simulink model "sampleModel305"  (R2021b)
settings: Solver=VariableStepAuto  StartTime=0.0  StopTime=10.0  RelTol=1e-3
libraries: simulink x7, slpidlib x1
settings Model: Creator=user  LastModifiedBy=user

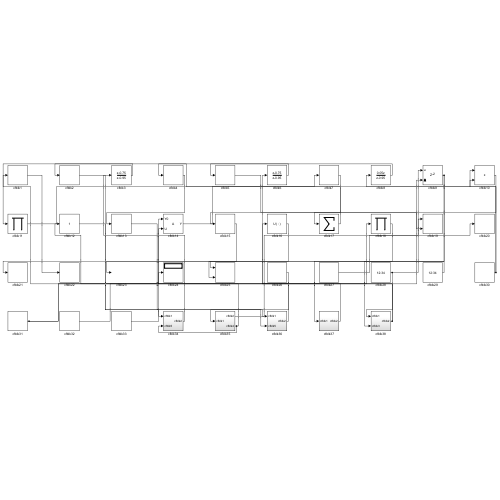
[thumbnail: Simulink's stored preview of the top-level diagram]
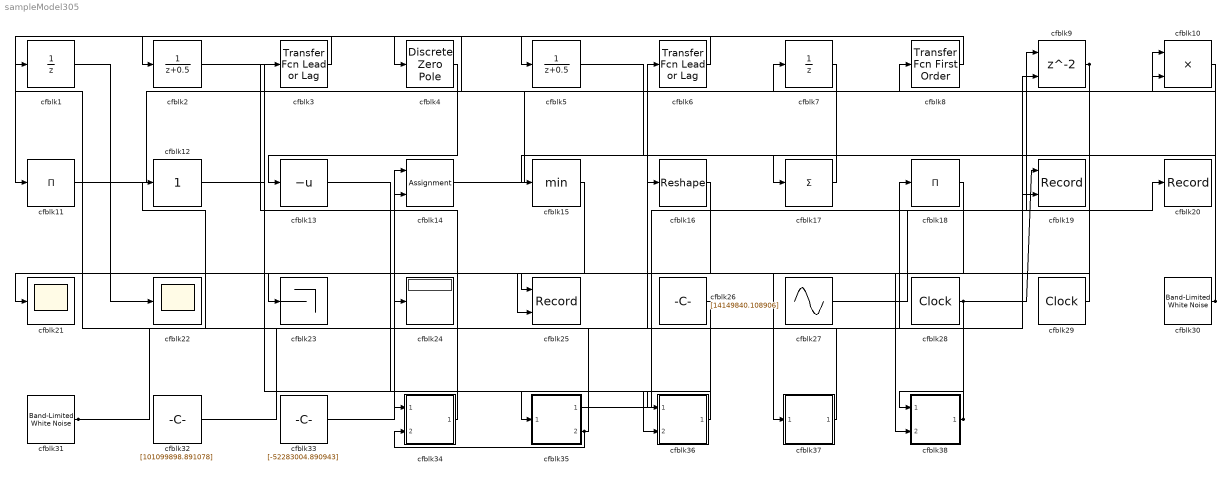
== system sampleModel305 ==
  cfblk1 : UnitDelay  HasFrameUpgradeWarning=on
  cfblk10 : Product  Inputs=**
  cfblk11 : Product  Inputs=*
  cfblk12 : simulink/Math Operations/Slider Gain  gain=1  low=0  high=2
  cfblk13 : UnaryMinus
  cfblk14 : Assignment  DiagnosticForDimensions=Warning  IndexOptions=Index vector (dialog)  Indices=1  OutputSizes=1
  cfblk15 : MinMax
  cfblk16 : Reshape
  cfblk17 : Sum  Inputs=+
  cfblk18 : Product  Inputs=*
  cfblk19 : Record  FileSettingsInternal="{\"entries\":[{\"content\":{\"excelSettings\":{\"content\":{},\"type\":\"Streamout.ExcelSettings\"}},\"type\":\"Streamout.FileSettingStorage\",\"uuid\":\"63984bb0-c559-4448-9fc6-104896ff0659\"}],\"packageUris\":[\"http://schema.mathworks.com/mf0/streamout_blocks/R2020a\"],\"version\":\"1.0\"}"  Layout=[1 1]  SignalsInternal="{\"entries\":[{\"content\":{\"signals\":[{\"content\":{\"blockPath\":[\"sampleModel305/cfblk19\"],\"channel\":[],\"dimensions\":[1],\"domain\":\"sampleModel305/cfblk19\",\"lineColor\":\"#a2142f\",\"plots\":[1],\"port\":1,\"sid\":[\"\"],\"signalID\":13014,\"signalName\":\"cfblk28\"},\"type\":\"RecordBlkView.Signal\",\"uuid\":\"141cd215-84be-4e50-999d-5b1fe4f06e84\"},{\"content\":{\"blockPath\":[\"sampleModel305/cfblk19\"],\"channel\":[],\"dimensions\":[1],\"domain\":\"sampleModel305/cfblk19\",\"lineColor\":\"#139fff\",\"plots\":[1],\"port\":2,\"sid\":[\"\"],\"signalID\":13018,\"signalName\":\"cfblk5\"},\"type\":\"RecordBlkView.Signal\",\"uuid\":\"dcc0499d-3265-4208-832f-2459034609dc\"}]},\"type\":\"RecordBlkView.InputSignals\",\"uuid\":\"7f0c9375-5767-4acb-9abc-590f8e22dae8\"}],\"packageUris\":[\"http://schema.mathworks.com/mf0/streamout_blocks/R2020a\"],\"version\":\"1.0\"}"  VisualizationBindings="{\"xyplotplugin\":{\"info\":[{\"series\":[{\"bindingParametersList\":[{\"parameter\":\"X-Axis\",\"signalID\":13014,\"signalName\":\"cfblk28\"},{\"parameter\":\"Y-Axis\",\"signalID\":13018,\"signalName\":\"cfblk5\"}],\"seriesID\":43943}],\"subplotID\":1}]}}"  CompatibilityTag=XY
  cfblk2 : DiscreteTransferFcn  SampleTime=1
  cfblk20 : Record  FileSettingsInternal="{\"entries\":[{\"content\":{\"excelSettings\":{\"content\":{},\"type\":\"Streamout.ExcelSettings\"}},\"type\":\"Streamout.FileSettingStorage\",\"uuid\":\"fa745143-092b-49d5-8c77-bd1d4f02d415\"}],\"packageUris\":[\"http://schema.mathworks.com/mf0/streamout_blocks/R2020a\"],\"version\":\"1.0\"}"  SignalsInternal="{\"entries\":[{\"content\":{\"signals\":[{\"content\":{\"blockPath\":[\"sampleModel305/cfblk20\"],\"channel\":[],\"dimensions\":[1],\"domain\":\"sampleModel305/cfblk20\",\"lineColor\":\"#7e2f8e\",\"plots\":[1],\"port\":1,\"sid\":[\"\"],\"signalID\":13030,\"signalName\":\"cfblk27\"},\"type\":\"RecordBlkView.Signal\",\"uuid\":\"72bc61b7-b3db-4e59-b8bd-afabd6830a11\"}]},\"type\":\"RecordBlkView.InputSignals\",\"uuid\":\"cfa96d27-1d36-46cd-bd3b-7bc137c001bd\"}],\"packageUris\":[\"http://schema.mathworks.com/mf0/streamout_blocks/R2020a\"],\"version\":\"1.0\"}"  VisualizationBindings="{\"sparklinesplugin\":{\"info\":[{\"bindingParametersList\":[],\"subplotID\":1}]}}"
  cfblk21 : Scope
  cfblk22 : Scope
  cfblk23 : Terminator
  cfblk24 : Display
  cfblk25 : Record  FileSettingsInternal="{\"entries\":[{\"content\":{\"excelSettings\":{\"content\":{},\"type\":\"Streamout.ExcelSettings\"}},\"type\":\"Streamout.FileSettingStorage\",\"uuid\":\"4ed7394e-1e80-4f63-a180-05586a1c6fb6\"}],\"packageUris\":[\"http://schema.mathworks.com/mf0/streamout_blocks/R2020a\"],\"version\":\"1.0\"}"  Layout=[1 1]  SignalsInternal="{\"entries\":[{\"content\":{\"signals\":[{\"content\":{\"blockPath\":[\"sampleModel305/cfblk25\"],\"channel\":[],\"dimensions\":[1],\"domain\":\"sampleModel305/cfblk25\",\"lineColor\":\"#a2142f\",\"plots\":[1],\"port\":1,\"sid\":[\"\"],\"signalID\":13022,\"signalName\":\"cfblk18\"},\"type\":\"RecordBlkView.Signal\",\"uuid\":\"0d41f3c0-332b-4af7-9193-0bd311ec3bc9\"},{\"content\":{\"blockPath\":[\"sampleModel305/cfblk25\"],\"channel\":[],\"dimensions\":[1],\"domain\":\"sampleModel305/cfblk25\",\"lineColor\":\"#139fff\",\"plots\":[1],\"port\":2,\"sid\":[\"\"],\"signalID\":13026,\"signalName\":\"cfblk16\"},\"type\":\"RecordBlkView.Signal\",\"uuid\":\"af7c6a5f-4348-43a5-9ee2-0d9b4d9b9d80\"}]},\"type\":\"RecordBlkView.InputSignals\",\"uuid\":\"7a96359f-dcc9-4f03-ae41-85340fe35594\"}],\"packageUris\":[\"http://schema.mathworks.com/mf0/streamout_blocks/R2020a\"],\"version\":\"1.0\"}"  VisualizationBindings="{\"xyplotplugin\":{\"info\":[{\"series\":[{\"bindingParametersList\":[{\"parameter\":\"X-Axis\",\"signalID\":13022,\"signalName\":\"cfblk18\"},{\"parameter\":\"Y-Axis\",\"signalID\":13026,\"signalName\":\"cfblk16\"}],\"seriesID\":33645}],\"subplotID\":1}]}}"  CompatibilityTag=XY
  cfblk26 : Constant  Value=[14149840.108906]  SampleTime=1
  cfblk27 : Sin  Amplitude=[654816307.615221]  Bias=[133220113.549446]  SampleTime=0
  cfblk28 : DigitalClock
  cfblk29 : DigitalClock
  cfblk3 : simulink/Discrete/Transfer Fcn Lead or Lag  PoleZ=0.95  ZeroZ=0.75  ICPrevOutput=0.0  ICPrevInput=0.0  DoSatur=off
      settings: SourceProductBaseCode=SL
  cfblk30 : simulink/Sources/Band-Limited White Noise  Cov=[4233247862.162008]  Ts=0.1  seed=[8090119593.000000]
  cfblk31 : simulink/Sources/Band-Limited White Noise  Cov=[2095450367.965964]  Ts=0.1  seed=[574629679.000000]
  cfblk32 : Constant  Value=[101099898.891078]  SampleTime=1
  cfblk33 : Constant  Value=[-52283004.890943]  SampleTime=1
  cfblk34 : Subsystem
  cfblk35 : Subsystem
  cfblk36 : Subsystem
  cfblk37 : Subsystem
  cfblk38 : Subsystem
  cfblk4 : DiscreteZeroPole  Poles=[0 0.5]  Gain=1
  cfblk5 : DiscreteTransferFcn  SampleTime=1
  cfblk6 : simulink/Discrete/Transfer Fcn Lead or Lag  PoleZ=0.95  ZeroZ=0.75  ICPrevOutput=0.0  ICPrevInput=0.0  DoSatur=off
      settings: SourceProductBaseCode=SL
  cfblk7 : UnitDelay  HasFrameUpgradeWarning=on
  cfblk8 : simulink/Discrete/Transfer Fcn First Order  PoleZ=0.95  ICPrevOutput=0.0  DoSatur=off
  cfblk9 : Delay  ShowEnablePort=on  SampleTime=1
      settings: InputPortMap=u0,e6
  wires:
  cfblk4/1 -> cfblk13/1
  cfblk17/1 -> cfblk4/1
  cfblk34/1(cfblk2) -> cfblk3/1
  cfblk3/1 -> cfblk11/1
  cfblk30/1 -> cfblk10/1, cfblk8/1
  cfblk35/1(cfblk2) -> cfblk9/1
  cfblk9/1 -> cfblk37/1(cfblk1), cfblk38/2(cfblk3)
  cfblk33/1 -> cfblk14/1
  cfblk8/1 -> cfblk5/1
  cfblk31/1 -> cfblk14/2, cfblk18/1
  cfblk37/1(cfblk2) -> cfblk6/1
  cfblk18/1 -> cfblk25/1
  cfblk36/1(cfblk2) -> cfblk1/1
  cfblk10/1 -> cfblk17/1
  cfblk14/1 -> cfblk10/2
  cfblk1/1 -> cfblk22/1
  cfblk35/2(cfblk4) -> cfblk24/1, cfblk34/2(cfblk5)
  cfblk26/1 -> cfblk35/1(cfblk1)
  cfblk28/1 -> cfblk19/1, cfblk38/1(cfblk1)
  cfblk15/1 -> cfblk21/1
  cfblk2/1 -> cfblk36/1(cfblk1)
  cfblk13/1 -> cfblk36/2(cfblk5)
  cfblk7/1 -> cfblk15/1
  cfblk38/1(cfblk2) -> cfblk16/1, cfblk12/1
  cfblk32/1 -> cfblk9/2
  cfblk12/1 -> cfblk34/1(cfblk1)
  cfblk5/1 -> cfblk19/2
  cfblk16/1 -> cfblk25/2
  cfblk29/1 -> cfblk23/1
  cfblk27/1 -> cfblk20/1
  cfblk11/1 -> cfblk7/1
  cfblk6/1 -> cfblk2/1

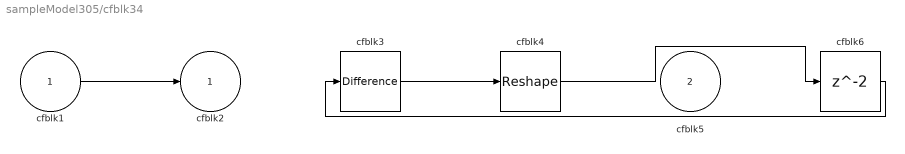
== system sampleModel305/cfblk34 ==
  cfblk1 : Inport
  cfblk5 : Inport  Port=2
  cfblk3 : simulink/Discrete/Difference  ICPrevInput=0.0  OutMin=[]  OutMax=[]  OutDataTypeStr=Inherit: Inherit via back propagation  OutDataType=fixdt(1, 16)  OutScaling=2^-10  DoSatur=off
  cfblk4 : Reshape
  cfblk6 : Delay  SampleTime=1
  cfblk2 : Outport
  wires:
  cfblk3/1 -> cfblk4/1
  cfblk1/1 -> cfblk2/1
  cfblk4/1 -> cfblk6/1
  cfblk6/1 -> cfblk3/1

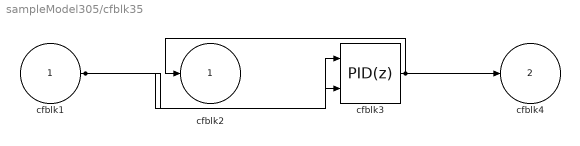
== system sampleModel305/cfblk35 ==
  cfblk1 : Inport
  cfblk3 : slpidlib/PID Controller (2DOF)  Controller=PID  Form=Parallel  TimeDomain=Discrete-time  UseExternalTs=off  SampleTime=1  IntegratorMethod=Forward Euler  FilterMethod=Forward Euler  ControllerParametersSource=internal  P=1  I=1  D=0  UseFilter=on  N=100  b=1  c=1  TunerSelectOption=Transfer Function Based (PID Tuner App)  InitialConditionSource=internal  InitialConditionForIntegrator=0  InitialConditionForFilter=0  DifferentiatorICPrevScaledInput=0  ExternalReset=none  TrackingMode=off  Kt=1  LimitOutput=off  SatLimitsSource=internal  UpperSaturationLimit=inf  LowerSaturationLimit=-inf  LinearizeAsGain=off  AntiWindupMode=none  Kb=1  POutMin=[]  POutMax=[]  IOutMin=[]  IOutMax=[]  DOutMin=[]  DOutMax=[]  NOutMin=[]  NOutMax=[]  bOutMin=[]  bOutMax=[]  cOutMin=[]  cOutMax=[]  SumOutMin=[]  SumOutMax=[]  SaturationOutMin=[]  SaturationOutMax=[]  PParamMin=[]  PParamMax=[]  IParamMin=[]  IParamMax=[]  DParamMin=[]  DParamMax=[]  NParamMin=[]  NParamMax=[]  bParamMin=[]  bParamMax=[]  cParamMin=[]  cParamMax=[]  KbParamMin=[]  KbParamMax=[]  KtParamMin=[]  KtParamMax=[]  KbOutMin=[]  KbOutMax=[]  KtOutMin=[]  KtOutMax=[]  IntegratorOutMin=[]  IntegratorOutMax=[]  FilterOutMin=[]  FilterOutMax=[]  SumI1OutMin=[]  SumI1OutMax=[]  SumI2OutMin=[]  SumI2OutMax=[]  SumI3OutMin=[]  SumI3OutMax=[]  SumI4OutMin=[]  SumI4OutMax=[]  SumDOutMin=[]  SumDOutMax=[]  Sum1OutMin=[]  Sum1OutMax=[]  Sum2OutMin=[]  Sum2OutMax=[]  Sum3OutMin=[]  Sum3OutMax=[]  DifferentiatorOutMin=[]  DifferentiatorOutMax=[]  FilterDiffOutCoefMin=[]  FilterDiffOutCoefMax=[]  ReciprocalOutMin=[]  ReciprocalOutMax=[]  SumDenOutMin=[]  SumDenOutMax=[]  SumNumOutMin=[]  SumNumOutMax=[]  DivideOutMin=[]  DivideOutMax=[]  UdiffTsProdOutMin=[]  UdiffTsProdOutMax=[]  NTsProdOutMin=[]  NTsProdOutMax=[]  UintegralTsProdOutMin=[]  UintegralTsProdOutMax=[]  UngainTsProdOutMin=[]  UngainTsProdOutMax=[]  IntegratorContinuousStateAttributes=''  IntegratorStateMustResolveToSignalObject=off  IntegratorRTWStateStorageClass=Auto  FilterContinuousStateAttributes=''  FilterStateMustResolveToSignalObject=off  FilterRTWStateStorageClass=Auto  ParallelPVariant=InternalParameters  IdealPVariant=Disabled  IVariant=InternalParameters  DVariant=InternalParameters  bVariant=InternalParameters  cVariant=InternalParameters  IntegratorVariant=Discrete  SatVariant=Disabled  AWVariant=Passthrough  PCopyVariant=Disabled  TRVariant=Disabled  FdbkBlocksVariant=Forward  IdealPFdbkVariant=Disabled  SatFdbkVariant=Disabled  DerivativeFilterVariant=ForwardEulerFilter  NVariant=InternalParameters  NCopyVariant=Disabled  FilterICVariant=InternalICsFilter  IntegratorICVariant=InternalICs  ExternalResetVariant=Disabled  TRSumVariant=Passthrough  SumFdbkVariant=Disabled  SumVariant=Sum_PID  TsampFilterVariant=InternalTs  TsampNgainVariant=Passthrough  TsampIntegralVariant=Passthrough  ExternalSaturationOutDataTypeStr=Inherit: Same as second input
      settings: SourceProductBaseCode=SL
  cfblk2 : Outport
  cfblk4 : Outport  Port=2
  wires:
  cfblk3/1 -> cfblk2/1, cfblk4/1
  cfblk1/1 -> cfblk3/1, cfblk3/2

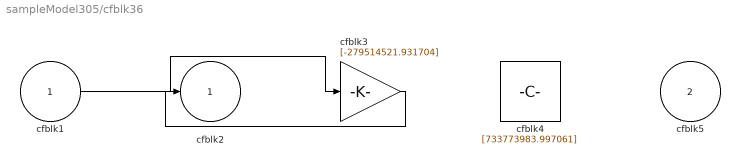
== system sampleModel305/cfblk36 ==
  cfblk1 : Inport
  cfblk5 : Inport  Port=2
  cfblk3 : Gain  Gain=[-279514521.931704]
  cfblk4 : Constant  Value=[733773983.997061]  SampleTime=1
  cfblk2 : Outport
  wires:
  cfblk1/1 -> cfblk3/1
  cfblk3/1 -> cfblk2/1

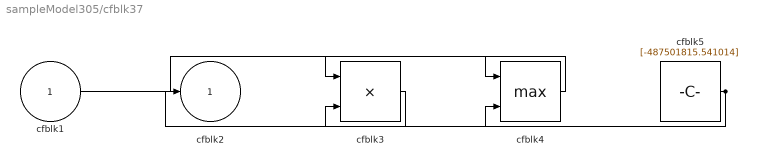
== system sampleModel305/cfblk37 ==
  cfblk1 : Inport
  cfblk3 : Product
  cfblk4 : MinMax  Function=max  Inputs=2
  cfblk5 : Constant  Value=[-487501815.541014]  SampleTime=1
  cfblk2 : Outport
  wires:
  cfblk1/1 -> cfblk4/1
  cfblk5/1 -> cfblk4/2, cfblk3/2
  cfblk4/1 -> cfblk3/1
  cfblk3/1 -> cfblk2/1

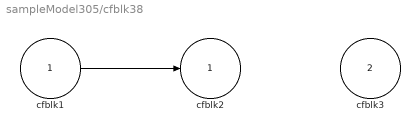
== system sampleModel305/cfblk38 ==
  cfblk1 : Inport
  cfblk3 : Inport  Port=2
  cfblk2 : Outport
  wires:
  cfblk1/1 -> cfblk2/1
